simulink model "ideal_bpsk_demodulator"  (R2013a)
settings: Solver=ode3  StartTime=0.0  StopTime=20/1200  FixedStep=(1/1200)/1024  RelTol=1e-3
libraries: commrandsrc2 x1, dsparch4 x1
settings Model: Creator=tibbs2010  LastModifiedBy=Cedric

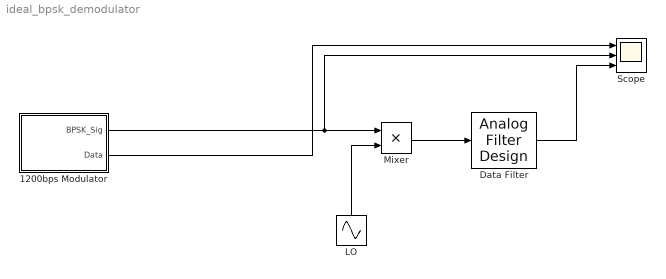
== system ideal_bpsk_demodulator ==
  1200bps Modulator : Subsystem
  Data Filter : dsparch4/Analog Filter Design  method=Butterworth  filttype=Lowpass  N=1  Wlo=2*pi*2400  Whi=80  Rp=2  Rs=40
  LO : Sin  Frequency=2*pi*1200  Samples=1024  SampleTime=(1/1200)/1024
  Mixer : Product
  Scope : Scope  NumInputPorts=3
      settings: YMin=-2~-2~-2  YMax=2~2~2
  wires:
  1200bps Modulator/1(BPSK_Sig) -> Scope/2, Mixer/1
  LO/1 -> Mixer/2
  Mixer/1 -> Data Filter/1
  Data Filter/1 -> Scope/3
  1200bps Modulator/2(Data) -> Scope/1

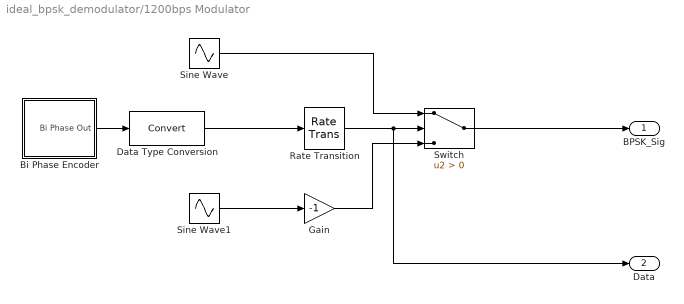
== system ideal_bpsk_demodulator/1200bps Modulator ==
  Bi Phase Encoder : Subsystem
  Data Type Conversion : DataTypeConversion
  Gain : Gain  Gain=-1
  Rate Transition : RateTransition
  Sine Wave : Sin  Frequency=2*pi*1200  Samples=1024  SampleTime=(1/1200)/1024
  Sine Wave1 : Sin  Frequency=2*pi*1200  Samples=1024  SampleTime=(1/1200)/1024
  Switch : Switch  Criteria=u2 > Threshold
  BPSK_Sig : Outport
  Data : Outport  Port=2
  wires:
  Switch/1 -> BPSK_Sig/1
  Bi Phase Encoder/1(Bi Phase Out) -> Data Type Conversion/1
  Rate Transition/1 -> Data/1, Switch/2
  Sine Wave/1 -> Switch/1
  Sine Wave1/1 -> Gain/1
  Gain/1 -> Switch/3
  Data Type Conversion/1 -> Rate Transition/1

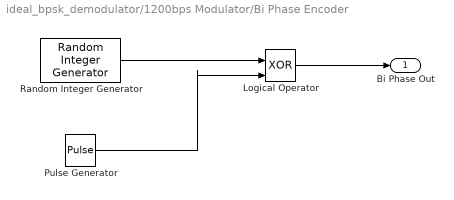
== system ideal_bpsk_demodulator/1200bps Modulator/Bi Phase Encoder ==
  Logical Operator : Logic  Operator=XOR  IconShape=distinctive  AllPortsSameDT=off  OutDataTypeStr=boolean
  Pulse Generator : DiscretePulseGenerator  Period=256  PulseWidth=128  SampleTime=1/(1200*1024)
  Random Integer Generator : commrandsrc2/Random Integer Generator  mul=2  seed=randseed  Ts=1/1200  frameBased=off  sampPerFrame=1  orient=off  outDataType=double
  Bi Phase Out : Outport
  wires:
  Pulse Generator/1 -> Logical Operator/2
  Logical Operator/1 -> Bi Phase Out/1
  Random Integer Generator/1 -> Logical Operator/1
